simulink model "Wiimote_test"  (Simulink 7.0)
settings: Solver=ode45  StartTime=0  StopTime=inf  FixedStep=0.005  RelTol=1e-3
libraries: quarc_library x1, simulink x1
settings Model: Creator=colinlea  LastModifiedBy=colinlea  ExtModeTrigDuration=10000
settings SolverCC: PositivePriorityOrder=on
settings RTWCC: SystemTargetFile=quarc_windows.tlc  TemplateMakefile=quarc_default_tmf  Description=QuaRC Win32 Target  ProcessScript=quarc_windows_make_rtw_hook
settings STFCustomTargetCC: TargetPreCompLibLocation=C:\DOCUME~1\ALLUSE~1\APPLIC~1\QuaRC\lib\2007b\windows\release  GenFloatMathFcnCalls=ANSI_C  SystemTargetFile=quarc_windows.tlc
settings GRTTargetCC: TargetPreCompLibLocation=C:\DOCUME~1\ALLUSE~1\APPLIC~1\QuaRC\lib\2007b\windows\release  CompOptLevelCompliant=off  MatFileLogging=off  ExtMode=on  ExtModeMexFile=quarc_comm

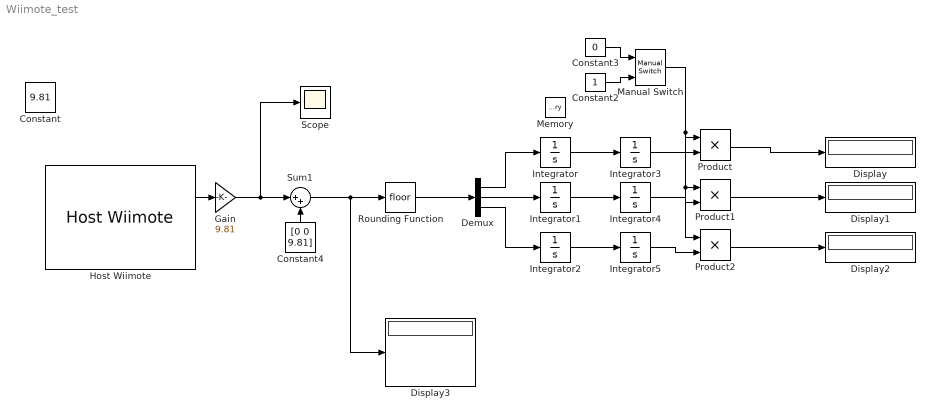
== system Wiimote_test ==
  Constant2 : Constant  OutDataType=sfix(16)  OutScaling=2^0
  Constant3 : Constant  Value=0  OutDataType=sfix(16)  OutScaling=2^0
  Constant4 : Constant  Orientation=up  Value=[0 0 9.81]  OutDataType=sfix(16)  OutScaling=2^0
  Demux : Demux  Outputs=3
  Display{,1..3} (4 alike) : Display
      Display3 settings: Decimation=3
  Gain : Gain  Gain=9.81  ParameterDataType=sfix(16)  ParameterScaling=2^0  OutDataType=sfix(16)  OutScaling=2^0
  Host Wiimote : quarc_library/Devices/Third-Party/Nintendo/Controllers/Host Wiimote  wiimote_number=0  sample_time=qc_get_step_size  buttons=[-1 0 0 0 0 0 0 0 0 0]  accel=[0 0 0]
  Integrator{,1..5} (6 alike) : Integrator
  Manual Switch : simulink/Signal Routing/Manual Switch  SystemSampleTime=-1  sw=0  action=0  varsize=off
  Memory : Memory  Orientation=left
  Product : Product  OutDataType=sfix(16)  OutScaling=2^0  RndMeth=Zero
  Product1 : Product  OutDataType=sfix(16)  OutScaling=2^0  RndMeth=Zero
  Product2 : Product  OutDataType=sfix(16)  OutScaling=2^0  RndMeth=Zero
  Rounding Function : Rounding
  Scope : Scope
      settings: YMin=-10  YMax=10  SaveName=WiimoteData  DataFormat=Array
  Sum1 : Sum  Inputs=|++  OutDataType=sfix(16)  OutScaling=2^0
  Constant : Constant  IOType=siggen  Value=9.81  OutDataType=sfix(16)  OutScaling=2^0
  wires:
  Host Wiimote/2 -> Gain/1
  Demux/1 -> Integrator/1
  Demux/2 -> Integrator1/1
  Integrator/1 -> Integrator3/1
  Integrator1/1 -> Integrator4/1
  Constant3/1 -> Manual Switch/1
  Constant2/1 -> Manual Switch/2
  Constant4/1 -> Sum1/2
  Gain/1 -> Sum1/1, Scope/1
  Sum1/1 -> Display3/1, Rounding Function/1
  Integrator3/1 -> Product/2
  Product2/1 -> Display2/1
  Product1/1 -> Display1/1
  Integrator5/1 -> Product2/2
  Manual Switch/1 -> Product/1, Product1/1, Product2/1
  Integrator4/1 -> Product1/2
  Demux/3 -> Integrator2/1
  Integrator2/1 -> Integrator5/1
  Rounding Function/1 -> Demux/1
  Product/1 -> Display/1
